simulink model "Supersonic_Heading_Autopilot"  (R2020a)
settings: Solver=VariableStepAuto  StartTime=0.0  StopTime=30  RelTol=1e-3
undefined symbols (not defined in the file or in its folder): A, B, C, D, g, u0
settings Model: Creator=AHSAN  LastModifiedBy=AHSAN

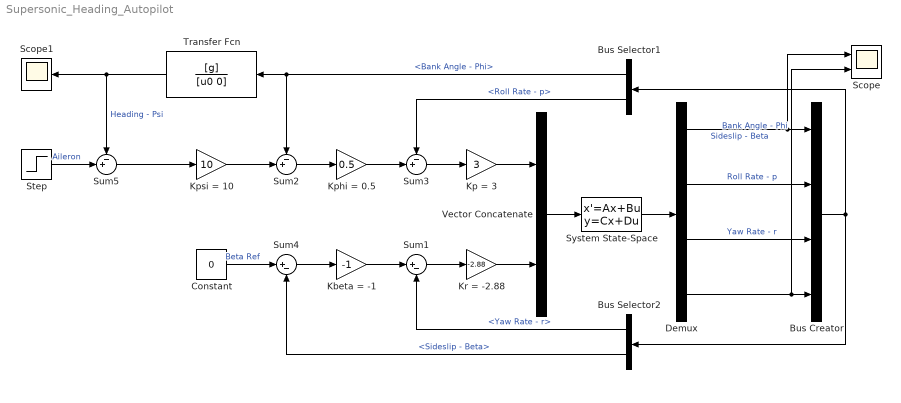
== system Supersonic_Heading_Autopilot ==
  Bus Creator : BusCreator  Inputs=4
  Bus Selector1 : BusSelector  OutputSignals=Bank Angle - Phi,Roll Rate - p
  Bus Selector2 : BusSelector  OutputSignals=Yaw Rate - r,Sideslip - Beta
  Constant : Constant  Value=0
  Demux : Demux
  Kbeta = -1 : Gain  Gain=-1
  Kp = 3 : Gain  Gain=3
  Kphi = 0.5 : Gain  Gain=0.5
  Kpsi = 10 : Gain  Gain=10
  Kr = -2.88 : Gain  Gain=-2.88
  Scope : Scope  NumInputPorts=2
  Scope1 : Scope
  Step : Step  Time=0  SampleTime=0
  Sum1 : Sum  Inputs=|+-
  Sum2 : Sum  Inputs=-+|
  Sum3 : Sum  Inputs=-+|
  Sum4 : Sum  Inputs=|+-
  Sum5 : Sum  Inputs=-+|
  System State-Space : StateSpace  A=A  B=B  C=C  D=D  InitialCondition=0
  Transfer Fcn : TransferFcn  Numerator=[g]  Denominator=[u0 0]
  Vector Concatenate : Concatenate
  wires:
  Constant/1 -> Sum4/1  "Beta Ref"
  Bus Creator/1 -> Bus Selector2/1, Bus Selector1/1
  Sum4/1 -> Kbeta = -1/1
  Bus Selector2/1 -> Sum1/2  "<Yaw Rate - r>"
  Kphi = 0.5/1 -> Sum3/2
  Demux/4 -> Scope/2, Bus Creator/4  "Bank Angle - Phi"
  Demux/2 -> Bus Creator/2  "Roll Rate - p"
  Demux/1 -> Scope/1, Bus Creator/1  "Sideslip - Beta"
  Demux/3 -> Bus Creator/3  "Yaw Rate - r"
  Sum1/1 -> Kr = -2.88/1
  Bus Selector2/2 -> Sum4/2  "<Sideslip - Beta>"
  Sum3/1 -> Kp = 3/1
  Kp = 3/1 -> Vector Concatenate/1
  System State-Space/1 -> Demux/1
  Transfer Fcn/1 -> Scope1/1, Sum5/1  "Heading - Psi"
  Vector Concatenate/1 -> System State-Space/1
  Bus Selector1/2 -> Sum3/1  "<Roll Rate - p>"
  Sum2/1 -> Kphi = 0.5/1
  Bus Selector1/1 -> Transfer Fcn/1, Sum2/1  "<Bank Angle - Phi>"
  Kbeta = -1/1 -> Sum1/1
  Kpsi = 10/1 -> Sum2/2
  Kr = -2.88/1 -> Vector Concatenate/2
  Step/1 -> Sum5/2  "Aileron"
  Sum5/1 -> Kpsi = 10/1
